simulink model "test_fft"  (R2012b)
settings: Solver=ode45  StartTime=0.0  StopTime=10.0  RelTol=1e-3
libraries: xbsIndex_r4 x6538, casper_library_misc x220, casper_library_delays x31, xbsReplacements_r4 x4, casper_library_ffts_twiddle x2, simulink x1
(part 95 of 104)

== system test_fft/fft0/fft_biplex_real_4x1/biplex_core/fft_stage_10/butterfly_direct/twiddle_general_4mult/coeff_gen ==
  rst : Inport
  Counter : xbsIndex_r4/Counter  cnt_type=Free Running  cnt_to=Inf  operation=Up  start_count=0  cnt_by_val=1  arith_type=Unsigned  n_bits=11  bin_pt=0  load_pin=off  rst=on  en=off  explicit_period=on  period=1  dbl_ovrd=off  use_behavioral_HDL=off  implementation=Fabric  block_type=counter
  ROM : xbsIndex_r4/ROM  depth=512  initVector="[1                                      0                     0.7071075439453125                    -0.7071075439453125                     0.9238739013671875                       -0.3826904296875                        0.3826904296875                    -0.9238739013671875                     0.9807891845703125                    -0.1950836181640625                      0.555572509765625                    -0.8314666748046875                     0.8314666748046875                     -0.555572509765625                     0.1950836181640625                    -0.9807891845703125                       0.99517822265625                       -0.0980224609375                        0.6343994140625                      -0.77301025390625                      0.881927490234375                    -0.4713897705078125                         0.290283203125                     -0.956939697265625                      0.956939697265625                        -0.290283203125                     0.4713897705078125                     -0.881927490234375                       0.77301025390625                       -0.6343994140625                        0.0980224609375                      -0.99517822265625                     0.9987945556640625                        -0.049072265625                     0.6715545654296875                    -0.7409515380859375                       0.90399169921875                      -0.42755126953125                      0.336883544921875                    -0.9415435791015625                       0.97003173828125                      -0.24298095703125                       0.51409912109375                      -0.85772705078125                     0.8032073974609375                           -0.595703125                         0.146728515625                    -0.9891815185546875                     0.9891815185546875                        -0.146728515625                            0.595703125                    -0.8032073974609375                       0.85772705078125                      -0.51409912109375                       0.24298095703125                      -0.97003173828125                     0.9415435791015625                     -0.336883544921875                       0.42755126953125                      -0.90399169921875                     0.7409515380859375                    -0.6715545654296875                         0.049072265625                    -0.9987945556640625                       0.99969482421875                       -0.0245361328125                      0.689544677734375                       -0.7242431640625                      0.914215087890625                     -0.405242919921875                      0.359893798828125                    -0.9329986572265625                        0.9757080078125                    -0.2191009521484375                      0.535003662109375                       -0.8448486328125                     0.8175811767578125                       -0.5758056640625                       0.17095947265625                    -0.9852752685546875                     0.9924774169921875                     -0.122406005859375                            0.615234375                    -0.7883453369140625                      0.870086669921875                    -0.4929046630859375                     0.2667083740234375                     -0.963775634765625                       0.94952392578125                    -0.3136749267578125                      0.449615478515625                     -0.893218994140625                        0.7572021484375                     -0.653167724609375                     0.0735626220703125                     -0.997283935546875                      0.997283935546875                    -0.0735626220703125                      0.653167724609375                       -0.7572021484375                      0.893218994140625                     -0.449615478515625                     0.3136749267578125 ...(+15932 chars)]"  distributed_mem=Block RAM  rst=off  init_reg=0  en=off  latency=4  gui_display_data_type=Fixed-point  arith_type="Signed  (2's comp)"  n_bits=18  bin_pt=16  preci_type=Single  exp_width=8  frac_width=24  dbl_ovrd=off  optimize=Area  use_rpm=on  block_type=sprom
  ROM1 : xbsIndex_r4/ROM  depth=512  initVector="[0                                     -1                    -0.7071075439453125                    -0.7071075439453125                       -0.3826904296875                    -0.9238739013671875                    -0.9238739013671875                       -0.3826904296875                    -0.1950836181640625                    -0.9807891845703125                    -0.8314666748046875                     -0.555572509765625                     -0.555572509765625                    -0.8314666748046875                    -0.9807891845703125                    -0.1950836181640625                       -0.0980224609375                      -0.99517822265625                      -0.77301025390625                       -0.6343994140625                    -0.4713897705078125                     -0.881927490234375                     -0.956939697265625                        -0.290283203125                        -0.290283203125                     -0.956939697265625                     -0.881927490234375                    -0.4713897705078125                       -0.6343994140625                      -0.77301025390625                      -0.99517822265625                       -0.0980224609375                        -0.049072265625                    -0.9987945556640625                    -0.7409515380859375                    -0.6715545654296875                      -0.42755126953125                      -0.90399169921875                    -0.9415435791015625                     -0.336883544921875                      -0.24298095703125                      -0.97003173828125                      -0.85772705078125                      -0.51409912109375                           -0.595703125                    -0.8032073974609375                    -0.9891815185546875                        -0.146728515625                        -0.146728515625                    -0.9891815185546875                    -0.8032073974609375                           -0.595703125                      -0.51409912109375                      -0.85772705078125                      -0.97003173828125                      -0.24298095703125                     -0.336883544921875                    -0.9415435791015625                      -0.90399169921875                      -0.42755126953125                    -0.6715545654296875                    -0.7409515380859375                    -0.9987945556640625                        -0.049072265625                       -0.0245361328125                      -0.99969482421875                       -0.7242431640625                     -0.689544677734375                     -0.405242919921875                     -0.914215087890625                    -0.9329986572265625                     -0.359893798828125                    -0.2191009521484375                       -0.9757080078125                       -0.8448486328125                     -0.535003662109375                       -0.5758056640625                    -0.8175811767578125                    -0.9852752685546875                      -0.17095947265625                     -0.122406005859375                    -0.9924774169921875                    -0.7883453369140625                           -0.615234375                    -0.4929046630859375                     -0.870086669921875                     -0.963775634765625                    -0.2667083740234375                    -0.3136749267578125                      -0.94952392578125                     -0.893218994140625                     -0.449615478515625                     -0.653167724609375                       -0.7572021484375                     -0.997283935546875                    -0.0735626220703125                    -0.0735626220703125                     -0.997283935546875                       -0.7572021484375                     -0.653167724609375                     -0.449615478515625                     -0.893218994140625                      -0.94952392578125 ...(+15932 chars)]"  distributed_mem=Block RAM  rst=off  init_reg=0  en=off  latency=4  gui_display_data_type=Fixed-point  arith_type="Signed  (2's comp)"  n_bits=18  bin_pt=16  preci_type=Single  exp_width=8  frac_width=24  dbl_ovrd=off  optimize=Area  use_rpm=on  block_type=sprom
  Slice : xbsIndex_r4/Slice  nbits=9  boolean_output=off  mode=Upper Bit Location + Width  bit1=0  base1=MSB of Input  bit0=0  base0=LSB of Input  dbl_ovrd=off  block_type=slice
  ri_to_c : casper_library_misc/ri_to_c
  w : Outport
  wires:
  ri_to_c/1 -> w/1
  rst/1 -> Counter/1
  Counter/1 -> Slice/1
  Slice/1 -> ROM/1, ROM1/1
  ROM/1 -> ri_to_c/1
  ROM1/1 -> ri_to_c/2

== system test_fft/fft0/fft_biplex_real_4x1/biplex_core/fft_stage_11/butterfly_direct/convert_of0/convert ==
  note: (ones_bit & 1) -> round-to-even
      | (ones_bit ^ 1) -> round-to-odd
      | (sign_bit & 1)-> round-to-zero
      | (sign_bit ^ 1) -> round-to-inf
      | (X ~| 1) -> round half down
      | (X | 1) -> round half up
  in : Inport
  Concat : xbsIndex_r4/Concat  num_inputs=2  dbl_ovrd=off  block_type=concat
      settings: block_version=10.1.3
  Constant : xbsIndex_r4/Constant  const=1  gui_display_data_type=Fixed-point  arith_type=Unsigned  n_bits=1  bin_pt=0  preci_type=Single  exp_width=8  frac_width=24  explicit_period=off  period=1  equ=P=C  opselect=C  inp2=PCIN>>17  opr=+  inp1=P  carry=CIN  dbl_ovrd=off  block_type=constant
  Reinterpret : xbsIndex_r4/Reinterpret  force_arith_type=on  arith_type=Unsigned  force_bin_pt=on  bin_pt=0  block_type=reinterpret
      settings: infoedit="Changes signal type without altering the binary representation.   You can changed the signal between signed and unsigned, and relocate the binary point.<P><P>Hardware notes: In hardware this block costs nothing.<P><P>Example:  Suppose the input is 6 bits wide, signed, with 2 fractional bits, and the output is forced to unsigned with 0 fractional bits.  Then an input of -2.0 (1110.00 in binary 2's complement) becomes an output of 56 (111000 in binary)."  block_version=10.1.3
  adder : xbsIndex_r4/AddSub  mode=Addition  use_carryin=off  use_carryout=off  en=off  latency=2  precision=User Defined  arith_type="Signed  (2's comp)"  n_bits=18  bin_pt=17  quantization=Truncate  overflow=Wrap  dbl_ovrd=off  use_behavioral_HDL=on  hw_selection=Fabric  pipelined=on  use_rpm=on  block_type=addsub
      settings: xl_area=[0, 0, 0, 0, 0, 0, 0]  block_version=10.1.3
  almost_half : xbsIndex_r4/Constant  const=7  gui_display_data_type=Fixed-point  arith_type=Unsigned  n_bits=21  bin_pt=0  preci_type=Single  exp_width=8  frac_width=24  explicit_period=off  period=1  equ=P=C  opselect=C  inp2=PCIN>>17  opr=+  inp1=P  carry=CIN  dbl_ovrd=off  block_type=constant
  bit : xbsIndex_r4/Slice  nbits=1  boolean_output=off  mode=Lower Bit Location + Width  bit1=0  base1=MSB of Input  bit0=0  base0=MSB of Input  dbl_ovrd=off  block_type=slice
      settings: infoedit="Extracts a given range of bits from each input sample and presents it at the output.  The output type is ordinarily unsigned with binary point at zero, but can be Boolean when the slice is one bit wide.<P><P>Hardware notes: In hardware this block costs nothing."  block_version=10.1.3
  force1 : xbsIndex_r4/Reinterpret  force_arith_type=on  arith_type="Signed  (2's comp)"  force_bin_pt=on  bin_pt=21  block_type=reinterpret
      settings: infoedit="Changes signal type without altering the binary representation.   You can changed the signal between signed and unsigned, and relocate the binary point.<P><P>Hardware notes: In hardware this block costs nothing.<P><P>Example:  Suppose the input is 6 bits wide, signed, with 2 fractional bits, and the output is forced to unsigned with 0 fractional bits.  Then an input of -2.0 (1110.00 in binary 2's complement) becomes an output of 56 (111000 in binary)."  block_version=10.1.3
  force2 : xbsIndex_r4/Reinterpret  force_arith_type=off  arith_type="Signed  (2's comp)"  force_bin_pt=on  bin_pt=21  block_type=reinterpret
      settings: infoedit="Changes signal type without altering the binary representation.   You can changed the signal between signed and unsigned, and relocate the binary point.<P><P>Hardware notes: In hardware this block costs nothing.<P><P>Example:  Suppose the input is 6 bits wide, signed, with 2 fractional bits, and the output is forced to unsigned with 0 fractional bits.  Then an input of -2.0 (1110.00 in binary 2's complement) becomes an output of 56 (111000 in binary)."  block_version=10.1.3
  tweak_op : xbsIndex_r4/Logical  logical_function=XOR  inputs=2  en=off  latency=0  precision=Full  arith_type=Unsigned  n_bits=8  bin_pt=2  align_bp=on  dbl_ovrd=off  block_type=logical
      settings: xl_area=[0, 0, 0, 0, 0, 0, 0]
  out : Outport
  wires:
  tweak_op/1 -> Concat/2
  Constant/1 -> tweak_op/2
  bit/1 -> tweak_op/1
  almost_half/1 -> force2/1
  in/1 -> Reinterpret/1, bit/1
  Concat/1 -> force1/1
  Reinterpret/1 -> Concat/1
  force1/1 -> adder/1
  force2/1 -> adder/2
  adder/1 -> out/1
